simulink model "simulink_model"  (R2021a)
settings: Solver=VariableStepAuto  StartTime=0.0  StopTime=10.0  RelTol=1e-3
settings Model: Creator=JaekyungSong  LastModifiedBy=JaekyungSong

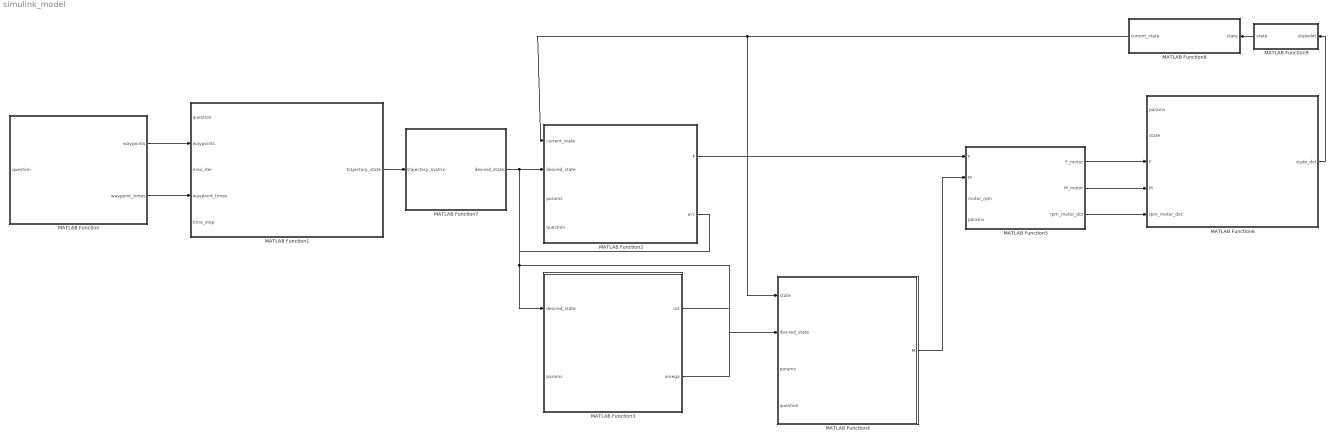
== system simulink_model ==
  MATLAB Function : MATLAB Function  TreatAsAtomicUnit=on
  MATLAB Function1 : MATLAB Function  TreatAsAtomicUnit=on
  MATLAB Function2 : MATLAB Function  TreatAsAtomicUnit=on
  MATLAB Function3 : MATLAB Function  TreatAsAtomicUnit=on
  MATLAB Function4 : MATLAB Function  TreatAsAtomicUnit=on
  MATLAB Function5 : MATLAB Function  TreatAsAtomicUnit=on
  MATLAB Function6 : MATLAB Function  TreatAsAtomicUnit=on
  MATLAB Function7 : MATLAB Function  TreatAsAtomicUnit=on
  MATLAB Function8 : MATLAB Function  TreatAsAtomicUnit=on
  MATLAB Function9 : MATLAB Function  TreatAsAtomicUnit=on
  wires:
  MATLAB Function/2(waypoint_times) -> MATLAB Function1/4(waypoint_times)
  MATLAB Function/1(waypoints) -> MATLAB Function1/2(waypoints)
  MATLAB Function1/1(trajectory_state) -> MATLAB Function7/1(trajectory_matrix)
  MATLAB Function7/1(desired_state) -> MATLAB Function4/2(desired_state), MATLAB Function3/1(desired_state), MATLAB Function2/2(desired_state)
  MATLAB Function2/2(acc) -> ?
  MATLAB Function3/1(rot) -> ?
  MATLAB Function3/2(omega) -> ?
  MATLAB Function2/1(F) -> MATLAB Function5/1(F)
  MATLAB Function4/1(M) -> MATLAB Function5/2(M)
  MATLAB Function5/3(rpm_motor_dot) -> MATLAB Function6/5(rpm_motor_dot)
  MATLAB Function5/2(M_motor) -> MATLAB Function6/4(M)
  MATLAB Function5/1(F_motor) -> MATLAB Function6/3(F)
  MATLAB Function9/1(state) -> MATLAB Function8/1(state)
  MATLAB Function6/1(state_dot) -> MATLAB Function9/1(statedot)
  MATLAB Function8/1(current_state) -> MATLAB Function4/1(state), MATLAB Function2/1(current_state)

== matlab function simulink_model/MATLAB Function1 ==
  data: question input; trajectory_state output; waypoints input; max_iter input; waypoint_times input; time_step input
function trajectory_state = trajectory_planner(question, waypoints, max_iter, waypoint_times, time_step)

% Input parameters
% 
%   question: Which question we are on in the assignment
%
%   waypoints: Series of points in [x; y; z; yaw] format
%
%   max_iter: Number of time steps
%
%   waypoint_times: Time we should be at each waypoint
%
%   time_step: Length of one time_step
%
% Output parameters
%
%   trajectory_sate: [15 x max_iter] output trajectory as a matrix of states:
%   [x; y; z; xdot; ydot; zdot; phi; theta; psi; phidot; thetadot; psidot; xacc; yacc; zacc];
%
%************  TRAJECTORY PLANNER ************************

% Write code here

% Sample code for hover trajectory
trajectory_state = zeros(15,max_iter);
% height of 15 for: [x; y; z; xdot; ydot; zdot; phi; theta; psi; phidot; thetadot; psidot; xacc; yacc; zacc];

current_waypoint_number = 1;

for iter = 1:max_iter
    if (current_waypoint_number<length(waypoint_times))
        if((iter*time_step)>waypoint_times(current_waypoint_number+1))
            current_waypoint_number = current_waypoint_number + 1;
        end
    end
        
    trajectory_state(1:3,iter) = waypoints(1:3,current_waypoint_number);
    trajectory_state(9,iter) = waypoints(4,current_waypoint_number);
    
end

end

== matlab function simulink_model/MATLAB Function ==
  data: question input; waypoints output; waypoint_times output
function [waypoints, waypoint_times] = lookup_waypoints(question)
%
% Input parameters
%
%   question: which question of the project we are on 
%      Possible arguments for question: 2, 3, 5, 6.2, 6.3, 6.5, 7, 9, 10
%
% Output parameters
%
%   waypoints: of the form [x; y; z; yaw]
% 
%   waypoint_times: [1 x n] vector of times where n is the number of waypoings, 
%   represents the seconds you should be at each respective waypoint
%
%************ LOOKUP WAYPOINTS ************************

% Write code here

%Sample waypoints for hover trajectory
if question == 2
    waypoints = [0 0.1 0.2 0.3; 0 0 0 0; 0.5 0.5 0.5 0.5; 0 0 0 0];
    waypoint_times = [0 2 4 6];

end

end

== matlab function simulink_model/MATLAB Function2 ==
  data: current_state input; F output; desired_state input; params input; question input; acc output
function [F, acc] = position_controller(current_state, desired_state, params, question)

% Input parameters
% 
%   current_state: The current state of the robot with the following fields:
%   current_state.pos = [x; y; z], 
%   current_state.vel = [x_dot; y_dot; z_dot],
%   current_state.rot = [phi; theta; psi], 
%   current_state.omega = [phidot; thetadot; psidot]
%   current_state.rpm = [w1; w2; w3; w4];
%
%   desired_state: The desired states are:
%   desired_state.pos = [x; y; z], 
%   desired_state.vel = [x_dot; y_dot; z_dot],
%   desired_state.rot = [phi; theta; psi], 
%   desired_state.omega = [phidot; thetadot; psidot]
%   desired_state.acc = [xdotdot; ydotdot; zdotdot];
%
%   params: Quadcopter parameters
%
%   question: Question number
%
% Output parameters
%
%   F: u1 or thrust
%
%   acc: will be stored as desired_state.acc = [xdotdot; ydotdot; zdotdot]
%
%************  POSITION CONTROLLER ************************

% Example PD gains
Kp1 = 17;
Kd1 = 6.6;

Kp2 = 17;
Kd2 = 6.6;

Kp3 = 20;
Kd3 = 9;

% Write code here

end

== matlab function simulink_model/MATLAB Function3 ==
  data: desired_state input; rot output; params input; omega output
function [rot, omega] = attitude_planner(desired_state, params)

% Input parameters
%
%   desired_state: The desired states are:
%   desired_state.pos = [x; y; z], 
%   desired_state.vel = [x_dot; y_dot; z_dot],
%   desired_state.rot = [phi; theta; psi], 
%   desired_state.omega = [phidot; thetadot; psidot]
%   desired_state.acc = [xdotdot; ydotdot; zdotdot];
%
%   params: Quadcopter parameters
%
% Output parameters
%
%   rot: will be stored as desired_state.rot = [phi; theta; psi], 
%
%   omega: will be stored as desired_state.omega = [phidot; thetadot; psidot]
%
%************  ATTITUDE PLANNER ************************

% Write code here

end

== matlab function simulink_model/MATLAB Function4 ==
  data: state input; M output; desired_state input; params input; question input
function M  = attitude_controller(state,desired_state,params,question)

% Input parameters
% 
%   current_state: The current state of the robot with the following fields:
%   current_state.pos = [x; y; z], 
%   current_state.vel = [x_dot; y_dot; z_dot],
%   current_state.rot = [phi; theta; psi], 
%   current_state.omega = [phidot; thetadot; psidot]
%   current_state.rpm = [w1; w2; w3; w4];
%
%   desired_state: The desired states are:
%   desired_state.pos = [x; y; z], 
%   desired_state.vel = [x_dot; y_dot; z_dot],
%   desired_state.rot = [phi; theta; psi], 
%   desired_state.omega = [phidot; thetadot; psidot]
%   desired_state.acc = [xdotdot; ydotdot; zdotdot];
%
%   params: Quadcopter parameters
%
%   question: Question number
%
% Output parameters
%
%   M: u2 or moment [M1; M2; M3]
%
%************  ATTITUDE CONTROLLER ************************

% Example PD gains
Kpphi = 190;
Kdphi = 30;

Kptheta = 198;
Kdtheta = 30;

Kppsi = 80;
Kdpsi = 17.88;

% Write code here

end

== matlab function simulink_model/MATLAB Function5 ==
  data: F input; F_motor output; M input; motor_rpm input; params input; M_motor output; rpm_motor_dot output
function [F_motor,M_motor,rpm_motor_dot] = motor_model(F,M,motor_rpm,params)

% Input parameters
% 
%   F,M: required force and moment
%
%   motor_rpm: current motor RPM
%
%   params: Quadcopter parameters
%
% Output parameters
%
%   F_motor: Actual thrust generated by Quadcopter's Motors
%
%   M_motor: Actual Moment generated by the Quadcopter's Motors
%
%   rpm_dot: Derivative of the RPM
%
%************ MOTOR MODEL ************************

% Write code here

end

== matlab function simulink_model/MATLAB Function6 ==
  data: params input; state_dot output; state input; F input; M input; rpm_motor_dot input
function state_dot  = dynamics(params, state, F, M, rpm_motor_dot)
% Input parameters
% 
%   state: current state, will be using ode45 to update
%
%   F, M: actual force and moment from motor model
%
%   rpm_motor_dot: actual change in RPM from motor model
% 
%   params: Quadcopter parameters
%
%   question: Question number
%
% Output parameters
%
%   state_dot: change in state
%
%************  DYNAMICS ************************

% Write code here
    
end

== matlab function simulink_model/MATLAB Function7 ==
  data: trajectory_matrix input; desired_state output
function desired_state = trj_mat_to_des_state(trajectory_matrix)

desired_state.pos = trajectory_matrix(1:3,iter);
desired_state.vel = trajectory_matrix(4:6,iter);
desired_state.rot = trajectory_matrix(7:9,iter);
desired_state.omega = trajectory_matrix(10:12,iter);
desired_state.acc = trajectory_matrix(13:15,iter);

== matlab function simulink_model/MATLAB Function8 ==
  data: state input; current_state output
function current_state = state_to_cur_state(state)
current_state.pos = state(1:3);
current_state.vel = state(4:6);
current_state.rot = state(7:9);
current_state.omega = state(10:12);
current_state.rpm = state(13:16);

== matlab function simulink_model/MATLAB Function9 ==
  data: statedot input; state output
function state = ode_solver(statedot)

state = statedot;
